simulink model "lab7p2"  (R2015a)
settings: Solver=ode45  StartTime=0.0  StopTime=160.0  RelTol=1e-3
libraries: simulink x3
settings Model: Creator=dg  LastModifiedBy=dg

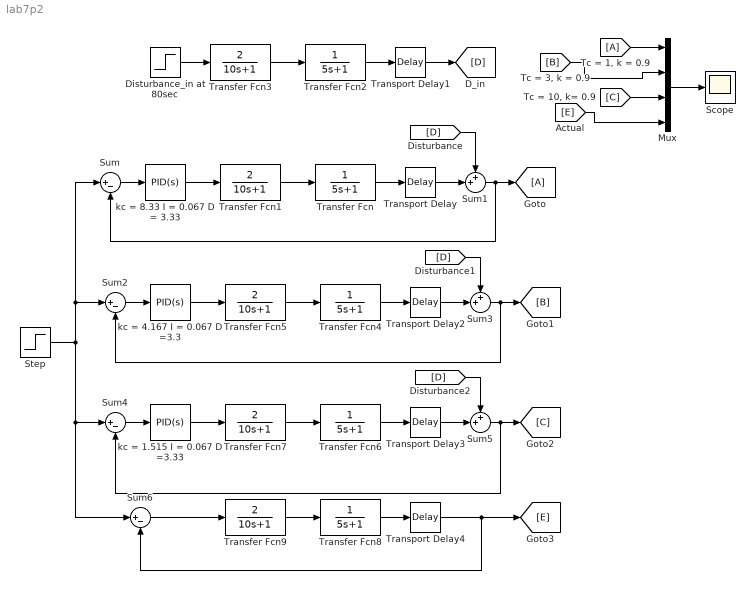
== system lab7p2 ==
  Disturbance_in at 80sec : Step  Time=80  SampleTime=0
  Mux : Mux
  Scope : Scope
      settings: ShowLegends=on
  Step : Step  SampleTime=0
  Sum{,2,4,6} (4 alike) : Sum  Inputs=|+-
  Sum1 : Sum  Inputs=++|
  Sum3 : Sum  Inputs=++|
  Sum5 : Sum  Inputs=++|
  Transfer Fcn{,2,4,6,8} (5 alike) : TransferFcn  Denominator=[5 1]
  Transfer Fcn{1,3,5,7,9} (5 alike) : TransferFcn  Numerator=[2]  Denominator=[10 1]
  Transport Delay{,1..4} (5 alike) : TransportDelay
  kc = 1.515 I = 0.067 D =3.33 : simulink/Continuous/PID Controller  Controller=PID  TimeDomain=Continuous-time  SampleTime=-1  IntegratorMethod=Forward Euler  FilterMethod=Forward Euler  Form=Ideal  UseFilter=on  ControllerParametersSource=internal  P=0.681  I=0.0667  D=3.33  N=100  InitialConditionSource=internal  InitialConditionForIntegrator=0  InitialConditionForFilter=0  ExternalReset=none  LimitOutput=off  UpperSaturationLimit=inf  LowerSaturationLimit=-inf  LinearizeAsGain=on  AntiWindupMode=none  Kb=1  TrackingMode=off  Kt=1  PParamMin=[]  PParamMax=[]  IParamMin=[]  IParamMax=[]  DParamMin=[]  DParamMax=[]  NParamMin=[]  NParamMax=[]  KbParamMin=[]  KbParamMax=[]  KtParamMin=[]  KtParamMax=[]  POutMin=[]  POutMax=[]  IOutMin=[]  IOutMax=[]  DOutMin=[]  DOutMax=[]  NOutMin=[]  NOutMax=[]  KbOutMin=[]  KbOutMax=[]  KtOutMin=[]  KtOutMax=[]  IntegratorOutMin=[]  IntegratorOutMax=[]  FilterOutMin=[]  FilterOutMax=[]  SumOutMin=[]  SumOutMax=[]  SumI1OutMin=[]  SumI1OutMax=[]  SumI2OutMin=[]  SumI2OutMax=[]  SumI3OutMin=[]  SumI3OutMax=[]  SumDOutMin=[]  SumDOutMax=[]  SaturationOutMin=[]  SaturationOutMax=[]  IntegratorContinuousStateAttributes=''  IntegratorStateMustResolveToSignalObject=off  IntegratorRTWStateStorageClass=Auto  FilterContinuousStateAttributes=''  FilterStateMustResolveToSignalObject=off  FilterRTWStateStorageClass=Auto  DifferentiatorICPrevScaledInput=0  DifferentiatorOutMin=[]  DifferentiatorOutMax=[]
  kc = 4.167 I = 0.067 D =3.3 : simulink/Continuous/PID Controller  Controller=PID  TimeDomain=Continuous-time  SampleTime=-1  IntegratorMethod=Forward Euler  FilterMethod=Forward Euler  Form=Ideal  UseFilter=on  ControllerParametersSource=internal  P=1.875  I=0.0667  D=3.33  N=100  InitialConditionSource=internal  InitialConditionForIntegrator=0  InitialConditionForFilter=0  ExternalReset=none  LimitOutput=off  UpperSaturationLimit=inf  LowerSaturationLimit=-inf  LinearizeAsGain=on  AntiWindupMode=none  Kb=1  TrackingMode=off  Kt=1  PParamMin=[]  PParamMax=[]  IParamMin=[]  IParamMax=[]  DParamMin=[]  DParamMax=[]  NParamMin=[]  NParamMax=[]  KbParamMin=[]  KbParamMax=[]  KtParamMin=[]  KtParamMax=[]  POutMin=[]  POutMax=[]  IOutMin=[]  IOutMax=[]  DOutMin=[]  DOutMax=[]  NOutMin=[]  NOutMax=[]  KbOutMin=[]  KbOutMax=[]  KtOutMin=[]  KtOutMax=[]  IntegratorOutMin=[]  IntegratorOutMax=[]  FilterOutMin=[]  FilterOutMax=[]  SumOutMin=[]  SumOutMax=[]  SumI1OutMin=[]  SumI1OutMax=[]  SumI2OutMin=[]  SumI2OutMax=[]  SumI3OutMin=[]  SumI3OutMax=[]  SumDOutMin=[]  SumDOutMax=[]  SaturationOutMin=[]  SaturationOutMax=[]  IntegratorContinuousStateAttributes=''  IntegratorStateMustResolveToSignalObject=off  IntegratorRTWStateStorageClass=Auto  FilterContinuousStateAttributes=''  FilterStateMustResolveToSignalObject=off  FilterRTWStateStorageClass=Auto  DifferentiatorICPrevScaledInput=0  DifferentiatorOutMin=[]  DifferentiatorOutMax=[]
  kc = 8.33 I = 0.067 D = 3.33 : simulink/Continuous/PID Controller  Controller=PID  TimeDomain=Continuous-time  SampleTime=-1  IntegratorMethod=Forward Euler  FilterMethod=Forward Euler  Form=Ideal  UseFilter=on  ControllerParametersSource=internal  P=8.33  I=0.0667  D=3.33  N=100  InitialConditionSource=internal  InitialConditionForIntegrator=0  InitialConditionForFilter=0  ExternalReset=none  LimitOutput=off  UpperSaturationLimit=inf  LowerSaturationLimit=-inf  LinearizeAsGain=on  AntiWindupMode=none  Kb=1  TrackingMode=off  Kt=1  PParamMin=[]  PParamMax=[]  IParamMin=[]  IParamMax=[]  DParamMin=[]  DParamMax=[]  NParamMin=[]  NParamMax=[]  KbParamMin=[]  KbParamMax=[]  KtParamMin=[]  KtParamMax=[]  POutMin=[]  POutMax=[]  IOutMin=[]  IOutMax=[]  DOutMin=[]  DOutMax=[]  NOutMin=[]  NOutMax=[]  KbOutMin=[]  KbOutMax=[]  KtOutMin=[]  KtOutMax=[]  IntegratorOutMin=[]  IntegratorOutMax=[]  FilterOutMin=[]  FilterOutMax=[]  SumOutMin=[]  SumOutMax=[]  SumI1OutMin=[]  SumI1OutMax=[]  SumI2OutMin=[]  SumI2OutMax=[]  SumI3OutMin=[]  SumI3OutMax=[]  SumDOutMin=[]  SumDOutMax=[]  SaturationOutMin=[]  SaturationOutMax=[]  IntegratorContinuousStateAttributes=''  IntegratorStateMustResolveToSignalObject=off  IntegratorRTWStateStorageClass=Auto  FilterContinuousStateAttributes=''  FilterStateMustResolveToSignalObject=off  FilterRTWStateStorageClass=Auto  DifferentiatorICPrevScaledInput=0  DifferentiatorOutMin=[]  DifferentiatorOutMax=[]
  wires:
  [A] -> Mux/1
  kc = 8.33 I = 0.067 D = 3.33/1 -> Transfer Fcn1/1
  Transfer Fcn1/1 -> Transfer Fcn/1
  Transfer Fcn/1 -> Transport Delay/1
  Sum/1 -> kc = 8.33 I = 0.067 D = 3.33/1
  Sum1/1 -> Sum/2, [A]
  [D] -> Sum1/1
  Transport Delay/1 -> Sum1/2
  Transfer Fcn3/1 -> Transfer Fcn2/1
  Transfer Fcn2/1 -> Transport Delay1/1
  Transport Delay1/1 -> [D]
  Disturbance_in at 80sec/1 -> Transfer Fcn3/1
  kc = 4.167 I = 0.067 D =3.3/1 -> Transfer Fcn5/1
  Transfer Fcn5/1 -> Transfer Fcn4/1
  Transfer Fcn4/1 -> Transport Delay2/1
  Sum2/1 -> kc = 4.167 I = 0.067 D =3.3/1
  Sum3/1 -> Sum2/2, [B]
  [D] -> Sum3/1
  Transport Delay2/1 -> Sum3/2
  kc = 1.515 I = 0.067 D =3.33/1 -> Transfer Fcn7/1
  Transfer Fcn7/1 -> Transfer Fcn6/1
  Transfer Fcn6/1 -> Transport Delay3/1
  Sum4/1 -> kc = 1.515 I = 0.067 D =3.33/1
  Sum5/1 -> Sum4/2, [C]
  [D] -> Sum5/1
  Transport Delay3/1 -> Sum5/2
  Step/1 -> Sum2/1, Sum/1, Sum6/1, Sum4/1
  Transfer Fcn9/1 -> Transfer Fcn8/1
  Transfer Fcn8/1 -> Transport Delay4/1
  Transport Delay4/1 -> [E], Sum6/2
  Sum6/1 -> Transfer Fcn9/1
  [B] -> Mux/2
  [C] -> Mux/3
  [E] -> Mux/4
  Mux/1 -> Scope/1
